simulink model "tensegrity_Val_like_sim_one_stage_v02"  (R2022b)
settings: Solver=ode15s  StartTime=0.0  StopTime=10  MaxStep=0.001  RelTol=1e-3
InitFcn:
  | tensegrity_Val_like_v02;
values from neighbouring files (symbols this model uses):
  a = 0.015    [parameters.m]
  A1 = [0.3, 0.3, 0.2]    [parameters_test_model.m]    (also in tensegrity_Val_like.m = [(G1+G2+G3)/3])
  A2 = [(G4+G5+G6)/3]    [tensegrity_Val_like.m]
  A3 = [(G7+G8+G9)/3]    [tensegrity_Val_like.m]
  A4 = [(B1+B2+B3)/3]    [tensegrity_Val_like.m]
  b_all = 2*ones(6, 1)    [parameters_test_model.m]
  F1 = [pos1(1), pos1(2), pos1(3)]    [parameters.m]
  F2 = [pos1(1)+dist, pos1(2), pos1(3)]    [parameters.m]
  F3 = [pos1(1)+dist/2, pos1(2)+dist, pos1(3)]    [parameters.m]
  F4 = [pos2(1), pos2(2), pos2(3)]    [parameters.m]
  F5 = [pos2(1)+dist, pos2(2), pos2(3)]    [parameters.m]
  F6 = [pos2(1)+dist/2, pos2(2)+dist, pos2(3)]    [parameters.m]
  F7 = [pos3(1), pos3(2), pos3(3)]    [parameters.m]
  F8 = [pos3(1)+dist, pos3(2), pos3(3)]    [parameters.m]
  F9 = [pos3(1)+dist/2, pos3(2)+dist, pos3(3)]    [parameters.m]
  k_all = 1e3*ones(6, 1)    [parameters_test_model.m]
  l = [0.08 0.08 0.08 0.15]'    [parameters.m]
  l0_all = [l01, l02, l03, l04, l05, l06]'    [parameters_test_model.m]
  lf = 0.05*ones(9, 1)    [parameters.m]
  predpeti = 0.95    [parameters_test_model.m]
undefined symbols (not defined in the file or in its folder): X, Y, Z
libraries: sm_lib x76, nesl_utility x73
(part 3 of 4)

== system tensegrity_Val_like_sim_one_stage_v02/internal cable force_19/cable force ==
  i : Inport
  Gain : Gain  Gain=predpeti
  PS-Simulink Converter1 : nesl_utility/PS-Simulink Converter  PhysicalDomain=network_engine_domain  SubClassName=ps_output  LeftPortType=input  RightPortType=output  PseudoPeriodic=off  Frequencies=[]  VectorFormat=1-D array  Unit=inherit  AffineConversion=off
  PS-Simulink Converter2 : nesl_utility/PS-Simulink Converter  PhysicalDomain=network_engine_domain  SubClassName=ps_output  LeftPortType=input  RightPortType=output  PseudoPeriodic=off  Frequencies=[]  VectorFormat=1-D array  Unit=inherit  AffineConversion=off
  Transform Sensor : sm_lib/Frames and Transforms/Transform Sensor  MeasurementFrame=World  SenseAngle=off  SenseAxis=off  SenseQ=off  SenseR=off  SenseRotationSequence=off  RotationSequence=XYX  SenseOmegaX=off  SenseOmegaY=off  SenseOmegaZ=off  SenseQDot=off  SenseRDot=off  SenseAlphaX=off  SenseAlphaY=off  SenseAlphaZ=off  SenseQDDot=off  SenseRDDot=off  SenseX=off  SenseY=off  SenseZ=off  SenseRad=off  SenseAzim=off  SenseDist=on  SenseInc=off  SenseXDot=off  SenseYDot=off  SenseZDot=off  SenseRadDot=off  SenseAzimDot=off  SenseDistDot=on  SenseIncDot=off  SenseXDDot=off  SenseYDDot=off  SenseZDDot=off  SenseRadDDot=off  SenseAzimDDot=off  SenseDistDDot=off  SenseIncDDot=off
  cable force computation : MATLAB Function  TreatAsAtomicUnit=on
  parameter selection : Subsystem
  TO : PMIOPort  Side=Right
  FROM : PMIOPort  Port=2  Side=Right
  Fc : Outport
  wires:
  Gain/1 -> cable force computation/3(l0)
  cable force computation/1(Fc) -> Fc/1
  parameter selection/2(b) -> cable force computation/2(b)
  parameter selection/3(l0) -> Gain/1
  parameter selection/1(k) -> cable force computation/1(k)
  PS-Simulink Converter1/1 -> cable force computation/4(l)
  PS-Simulink Converter2/1 -> cable force computation/5(v)
  i/1 -> parameter selection/1(i)
  connections:
  Transform Sensor/RConn3 -- PS-Simulink Converter2/LConn1
  Transform Sensor/RConn2 -- PS-Simulink Converter1/LConn1
  Transform Sensor/RConn1 -- TO/RConn1
  Transform Sensor/LConn1 -- FROM/RConn1

== system tensegrity_Val_like_sim_one_stage_v02/internal cable force_2/cable force ==
  i : Inport
  Gain : Gain  Gain=predpeti
  PS-Simulink Converter1 : nesl_utility/PS-Simulink Converter  PhysicalDomain=network_engine_domain  SubClassName=ps_output  LeftPortType=input  RightPortType=output  PseudoPeriodic=off  Frequencies=[]  VectorFormat=1-D array  Unit=inherit  AffineConversion=off
  PS-Simulink Converter2 : nesl_utility/PS-Simulink Converter  PhysicalDomain=network_engine_domain  SubClassName=ps_output  LeftPortType=input  RightPortType=output  PseudoPeriodic=off  Frequencies=[]  VectorFormat=1-D array  Unit=inherit  AffineConversion=off
  Transform Sensor : sm_lib/Frames and Transforms/Transform Sensor  MeasurementFrame=World  SenseAngle=off  SenseAxis=off  SenseQ=off  SenseR=off  SenseRotationSequence=off  RotationSequence=XYX  SenseOmegaX=off  SenseOmegaY=off  SenseOmegaZ=off  SenseQDot=off  SenseRDot=off  SenseAlphaX=off  SenseAlphaY=off  SenseAlphaZ=off  SenseQDDot=off  SenseRDDot=off  SenseX=off  SenseY=off  SenseZ=off  SenseRad=off  SenseAzim=off  SenseDist=on  SenseInc=off  SenseXDot=off  SenseYDot=off  SenseZDot=off  SenseRadDot=off  SenseAzimDot=off  SenseDistDot=on  SenseIncDot=off  SenseXDDot=off  SenseYDDot=off  SenseZDDot=off  SenseRadDDot=off  SenseAzimDDot=off  SenseDistDDot=off  SenseIncDDot=off
  cable force computation : MATLAB Function  TreatAsAtomicUnit=on
  parameter selection : Subsystem
  TO : PMIOPort  Side=Right
  FROM : PMIOPort  Port=2  Side=Right
  Fc : Outport
  wires:
  i/1 -> parameter selection/1(i)
  PS-Simulink Converter2/1 -> cable force computation/5(v)
  PS-Simulink Converter1/1 -> cable force computation/4(l)
  parameter selection/1(k) -> cable force computation/1(k)
  parameter selection/3(l0) -> Gain/1
  parameter selection/2(b) -> cable force computation/2(b)
  cable force computation/1(Fc) -> Fc/1
  Gain/1 -> cable force computation/3(l0)
  connections:
  Transform Sensor/LConn1 -- FROM/RConn1
  Transform Sensor/RConn1 -- TO/RConn1
  Transform Sensor/RConn2 -- PS-Simulink Converter1/LConn1
  Transform Sensor/RConn3 -- PS-Simulink Converter2/LConn1

== system tensegrity_Val_like_sim_one_stage_v02/internal cable force_20/cable force ==
  i : Inport
  Gain : Gain  Gain=predpeti
  PS-Simulink Converter1 : nesl_utility/PS-Simulink Converter  PhysicalDomain=network_engine_domain  SubClassName=ps_output  LeftPortType=input  RightPortType=output  PseudoPeriodic=off  Frequencies=[]  VectorFormat=1-D array  Unit=inherit  AffineConversion=off
  PS-Simulink Converter2 : nesl_utility/PS-Simulink Converter  PhysicalDomain=network_engine_domain  SubClassName=ps_output  LeftPortType=input  RightPortType=output  PseudoPeriodic=off  Frequencies=[]  VectorFormat=1-D array  Unit=inherit  AffineConversion=off
  Transform Sensor : sm_lib/Frames and Transforms/Transform Sensor  MeasurementFrame=World  SenseAngle=off  SenseAxis=off  SenseQ=off  SenseR=off  SenseRotationSequence=off  RotationSequence=XYX  SenseOmegaX=off  SenseOmegaY=off  SenseOmegaZ=off  SenseQDot=off  SenseRDot=off  SenseAlphaX=off  SenseAlphaY=off  SenseAlphaZ=off  SenseQDDot=off  SenseRDDot=off  SenseX=off  SenseY=off  SenseZ=off  SenseRad=off  SenseAzim=off  SenseDist=on  SenseInc=off  SenseXDot=off  SenseYDot=off  SenseZDot=off  SenseRadDot=off  SenseAzimDot=off  SenseDistDot=on  SenseIncDot=off  SenseXDDot=off  SenseYDDot=off  SenseZDDot=off  SenseRadDDot=off  SenseAzimDDot=off  SenseDistDDot=off  SenseIncDDot=off
  cable force computation : MATLAB Function  TreatAsAtomicUnit=on
  parameter selection : Subsystem
  TO : PMIOPort  Side=Right
  FROM : PMIOPort  Port=2  Side=Right
  Fc : Outport
  wires:
  i/1 -> parameter selection/1(i)
  PS-Simulink Converter2/1 -> cable force computation/5(v)
  PS-Simulink Converter1/1 -> cable force computation/4(l)
  parameter selection/1(k) -> cable force computation/1(k)
  parameter selection/3(l0) -> Gain/1
  parameter selection/2(b) -> cable force computation/2(b)
  cable force computation/1(Fc) -> Fc/1
  Gain/1 -> cable force computation/3(l0)
  connections:
  Transform Sensor/LConn1 -- FROM/RConn1
  Transform Sensor/RConn1 -- TO/RConn1
  Transform Sensor/RConn2 -- PS-Simulink Converter1/LConn1
  Transform Sensor/RConn3 -- PS-Simulink Converter2/LConn1

== system tensegrity_Val_like_sim_one_stage_v02/internal cable force_21/cable force ==
  i : Inport
  Gain : Gain  Gain=predpeti
  PS-Simulink Converter1 : nesl_utility/PS-Simulink Converter  PhysicalDomain=network_engine_domain  SubClassName=ps_output  LeftPortType=input  RightPortType=output  PseudoPeriodic=off  Frequencies=[]  VectorFormat=1-D array  Unit=inherit  AffineConversion=off
  PS-Simulink Converter2 : nesl_utility/PS-Simulink Converter  PhysicalDomain=network_engine_domain  SubClassName=ps_output  LeftPortType=input  RightPortType=output  PseudoPeriodic=off  Frequencies=[]  VectorFormat=1-D array  Unit=inherit  AffineConversion=off
  Transform Sensor : sm_lib/Frames and Transforms/Transform Sensor  MeasurementFrame=World  SenseAngle=off  SenseAxis=off  SenseQ=off  SenseR=off  SenseRotationSequence=off  RotationSequence=XYX  SenseOmegaX=off  SenseOmegaY=off  SenseOmegaZ=off  SenseQDot=off  SenseRDot=off  SenseAlphaX=off  SenseAlphaY=off  SenseAlphaZ=off  SenseQDDot=off  SenseRDDot=off  SenseX=off  SenseY=off  SenseZ=off  SenseRad=off  SenseAzim=off  SenseDist=on  SenseInc=off  SenseXDot=off  SenseYDot=off  SenseZDot=off  SenseRadDot=off  SenseAzimDot=off  SenseDistDot=on  SenseIncDot=off  SenseXDDot=off  SenseYDDot=off  SenseZDDot=off  SenseRadDDot=off  SenseAzimDDot=off  SenseDistDDot=off  SenseIncDDot=off
  cable force computation : MATLAB Function  TreatAsAtomicUnit=on
  parameter selection : Subsystem
  TO : PMIOPort  Side=Right
  FROM : PMIOPort  Port=2  Side=Right
  Fc : Outport
  wires:
  Gain/1 -> cable force computation/3(l0)
  cable force computation/1(Fc) -> Fc/1
  parameter selection/2(b) -> cable force computation/2(b)
  parameter selection/3(l0) -> Gain/1
  parameter selection/1(k) -> cable force computation/1(k)
  PS-Simulink Converter1/1 -> cable force computation/4(l)
  PS-Simulink Converter2/1 -> cable force computation/5(v)
  i/1 -> parameter selection/1(i)
  connections:
  Transform Sensor/RConn3 -- PS-Simulink Converter2/LConn1
  Transform Sensor/RConn2 -- PS-Simulink Converter1/LConn1
  Transform Sensor/RConn1 -- TO/RConn1
  Transform Sensor/LConn1 -- FROM/RConn1

== system tensegrity_Val_like_sim_one_stage_v02/internal cable force_22/cable force ==
  i : Inport
  Gain : Gain  Gain=predpeti
  PS-Simulink Converter1 : nesl_utility/PS-Simulink Converter  PhysicalDomain=network_engine_domain  SubClassName=ps_output  LeftPortType=input  RightPortType=output  PseudoPeriodic=off  Frequencies=[]  VectorFormat=1-D array  Unit=inherit  AffineConversion=off
  PS-Simulink Converter2 : nesl_utility/PS-Simulink Converter  PhysicalDomain=network_engine_domain  SubClassName=ps_output  LeftPortType=input  RightPortType=output  PseudoPeriodic=off  Frequencies=[]  VectorFormat=1-D array  Unit=inherit  AffineConversion=off
  Transform Sensor : sm_lib/Frames and Transforms/Transform Sensor  MeasurementFrame=World  SenseAngle=off  SenseAxis=off  SenseQ=off  SenseR=off  SenseRotationSequence=off  RotationSequence=XYX  SenseOmegaX=off  SenseOmegaY=off  SenseOmegaZ=off  SenseQDot=off  SenseRDot=off  SenseAlphaX=off  SenseAlphaY=off  SenseAlphaZ=off  SenseQDDot=off  SenseRDDot=off  SenseX=off  SenseY=off  SenseZ=off  SenseRad=off  SenseAzim=off  SenseDist=on  SenseInc=off  SenseXDot=off  SenseYDot=off  SenseZDot=off  SenseRadDot=off  SenseAzimDot=off  SenseDistDot=on  SenseIncDot=off  SenseXDDot=off  SenseYDDot=off  SenseZDDot=off  SenseRadDDot=off  SenseAzimDDot=off  SenseDistDDot=off  SenseIncDDot=off
  cable force computation : MATLAB Function  TreatAsAtomicUnit=on
  parameter selection : Subsystem
  TO : PMIOPort  Side=Right
  FROM : PMIOPort  Port=2  Side=Right
  Fc : Outport
  wires:
  Gain/1 -> cable force computation/3(l0)
  cable force computation/1(Fc) -> Fc/1
  parameter selection/2(b) -> cable force computation/2(b)
  parameter selection/3(l0) -> Gain/1
  parameter selection/1(k) -> cable force computation/1(k)
  PS-Simulink Converter1/1 -> cable force computation/4(l)
  PS-Simulink Converter2/1 -> cable force computation/5(v)
  i/1 -> parameter selection/1(i)
  connections:
  Transform Sensor/RConn3 -- PS-Simulink Converter2/LConn1
  Transform Sensor/RConn2 -- PS-Simulink Converter1/LConn1
  Transform Sensor/RConn1 -- TO/RConn1
  Transform Sensor/LConn1 -- FROM/RConn1

== system tensegrity_Val_like_sim_one_stage_v02/internal cable force_23/cable force ==
  i : Inport
  Gain : Gain  Gain=predpeti
  PS-Simulink Converter1 : nesl_utility/PS-Simulink Converter  PhysicalDomain=network_engine_domain  SubClassName=ps_output  LeftPortType=input  RightPortType=output  PseudoPeriodic=off  Frequencies=[]  VectorFormat=1-D array  Unit=inherit  AffineConversion=off
  PS-Simulink Converter2 : nesl_utility/PS-Simulink Converter  PhysicalDomain=network_engine_domain  SubClassName=ps_output  LeftPortType=input  RightPortType=output  PseudoPeriodic=off  Frequencies=[]  VectorFormat=1-D array  Unit=inherit  AffineConversion=off
  Transform Sensor : sm_lib/Frames and Transforms/Transform Sensor  MeasurementFrame=World  SenseAngle=off  SenseAxis=off  SenseQ=off  SenseR=off  SenseRotationSequence=off  RotationSequence=XYX  SenseOmegaX=off  SenseOmegaY=off  SenseOmegaZ=off  SenseQDot=off  SenseRDot=off  SenseAlphaX=off  SenseAlphaY=off  SenseAlphaZ=off  SenseQDDot=off  SenseRDDot=off  SenseX=off  SenseY=off  SenseZ=off  SenseRad=off  SenseAzim=off  SenseDist=on  SenseInc=off  SenseXDot=off  SenseYDot=off  SenseZDot=off  SenseRadDot=off  SenseAzimDot=off  SenseDistDot=on  SenseIncDot=off  SenseXDDot=off  SenseYDDot=off  SenseZDDot=off  SenseRadDDot=off  SenseAzimDDot=off  SenseDistDDot=off  SenseIncDDot=off
  cable force computation : MATLAB Function  TreatAsAtomicUnit=on
  parameter selection : Subsystem
  TO : PMIOPort  Side=Right
  FROM : PMIOPort  Port=2  Side=Right
  Fc : Outport
  wires:
  Gain/1 -> cable force computation/3(l0)
  cable force computation/1(Fc) -> Fc/1
  parameter selection/2(b) -> cable force computation/2(b)
  parameter selection/3(l0) -> Gain/1
  parameter selection/1(k) -> cable force computation/1(k)
  PS-Simulink Converter1/1 -> cable force computation/4(l)
  PS-Simulink Converter2/1 -> cable force computation/5(v)
  i/1 -> parameter selection/1(i)
  connections:
  Transform Sensor/RConn3 -- PS-Simulink Converter2/LConn1
  Transform Sensor/RConn2 -- PS-Simulink Converter1/LConn1
  Transform Sensor/RConn1 -- TO/RConn1
  Transform Sensor/LConn1 -- FROM/RConn1

== system tensegrity_Val_like_sim_one_stage_v02/internal cable force_3/cable force ==
  i : Inport
  Gain : Gain  Gain=predpeti
  PS-Simulink Converter1 : nesl_utility/PS-Simulink Converter  PhysicalDomain=network_engine_domain  SubClassName=ps_output  LeftPortType=input  RightPortType=output  PseudoPeriodic=off  Frequencies=[]  VectorFormat=1-D array  Unit=inherit  AffineConversion=off
  PS-Simulink Converter2 : nesl_utility/PS-Simulink Converter  PhysicalDomain=network_engine_domain  SubClassName=ps_output  LeftPortType=input  RightPortType=output  PseudoPeriodic=off  Frequencies=[]  VectorFormat=1-D array  Unit=inherit  AffineConversion=off
  Transform Sensor : sm_lib/Frames and Transforms/Transform Sensor  MeasurementFrame=World  SenseAngle=off  SenseAxis=off  SenseQ=off  SenseR=off  SenseRotationSequence=off  RotationSequence=XYX  SenseOmegaX=off  SenseOmegaY=off  SenseOmegaZ=off  SenseQDot=off  SenseRDot=off  SenseAlphaX=off  SenseAlphaY=off  SenseAlphaZ=off  SenseQDDot=off  SenseRDDot=off  SenseX=off  SenseY=off  SenseZ=off  SenseRad=off  SenseAzim=off  SenseDist=on  SenseInc=off  SenseXDot=off  SenseYDot=off  SenseZDot=off  SenseRadDot=off  SenseAzimDot=off  SenseDistDot=on  SenseIncDot=off  SenseXDDot=off  SenseYDDot=off  SenseZDDot=off  SenseRadDDot=off  SenseAzimDDot=off  SenseDistDDot=off  SenseIncDDot=off
  cable force computation : MATLAB Function  TreatAsAtomicUnit=on
  parameter selection : Subsystem
  TO : PMIOPort  Side=Right
  FROM : PMIOPort  Port=2  Side=Right
  Fc : Outport
  wires:
  Gain/1 -> cable force computation/3(l0)
  cable force computation/1(Fc) -> Fc/1
  parameter selection/2(b) -> cable force computation/2(b)
  parameter selection/3(l0) -> Gain/1
  parameter selection/1(k) -> cable force computation/1(k)
  PS-Simulink Converter1/1 -> cable force computation/4(l)
  PS-Simulink Converter2/1 -> cable force computation/5(v)
  i/1 -> parameter selection/1(i)
  connections:
  Transform Sensor/RConn3 -- PS-Simulink Converter2/LConn1
  Transform Sensor/RConn2 -- PS-Simulink Converter1/LConn1
  Transform Sensor/RConn1 -- TO/RConn1
  Transform Sensor/LConn1 -- FROM/RConn1

== system tensegrity_Val_like_sim_one_stage_v02/internal cable force_4/cable force ==
  i : Inport
  Gain : Gain  Gain=predpeti
  PS-Simulink Converter1 : nesl_utility/PS-Simulink Converter  PhysicalDomain=network_engine_domain  SubClassName=ps_output  LeftPortType=input  RightPortType=output  PseudoPeriodic=off  Frequencies=[]  VectorFormat=1-D array  Unit=inherit  AffineConversion=off
  PS-Simulink Converter2 : nesl_utility/PS-Simulink Converter  PhysicalDomain=network_engine_domain  SubClassName=ps_output  LeftPortType=input  RightPortType=output  PseudoPeriodic=off  Frequencies=[]  VectorFormat=1-D array  Unit=inherit  AffineConversion=off
  Transform Sensor : sm_lib/Frames and Transforms/Transform Sensor  MeasurementFrame=World  SenseAngle=off  SenseAxis=off  SenseQ=off  SenseR=off  SenseRotationSequence=off  RotationSequence=XYX  SenseOmegaX=off  SenseOmegaY=off  SenseOmegaZ=off  SenseQDot=off  SenseRDot=off  SenseAlphaX=off  SenseAlphaY=off  SenseAlphaZ=off  SenseQDDot=off  SenseRDDot=off  SenseX=off  SenseY=off  SenseZ=off  SenseRad=off  SenseAzim=off  SenseDist=on  SenseInc=off  SenseXDot=off  SenseYDot=off  SenseZDot=off  SenseRadDot=off  SenseAzimDot=off  SenseDistDot=on  SenseIncDot=off  SenseXDDot=off  SenseYDDot=off  SenseZDDot=off  SenseRadDDot=off  SenseAzimDDot=off  SenseDistDDot=off  SenseIncDDot=off
  cable force computation : MATLAB Function  TreatAsAtomicUnit=on
  parameter selection : Subsystem
  TO : PMIOPort  Side=Right
  FROM : PMIOPort  Port=2  Side=Right
  Fc : Outport
  wires:
  Gain/1 -> cable force computation/3(l0)
  cable force computation/1(Fc) -> Fc/1
  parameter selection/2(b) -> cable force computation/2(b)
  parameter selection/3(l0) -> Gain/1
  parameter selection/1(k) -> cable force computation/1(k)
  PS-Simulink Converter1/1 -> cable force computation/4(l)
  PS-Simulink Converter2/1 -> cable force computation/5(v)
  i/1 -> parameter selection/1(i)
  connections:
  Transform Sensor/RConn3 -- PS-Simulink Converter2/LConn1
  Transform Sensor/RConn2 -- PS-Simulink Converter1/LConn1
  Transform Sensor/RConn1 -- TO/RConn1
  Transform Sensor/LConn1 -- FROM/RConn1

== system tensegrity_Val_like_sim_one_stage_v02/internal cable force_5/cable force ==
  i : Inport
  Gain : Gain  Gain=predpeti
  PS-Simulink Converter1 : nesl_utility/PS-Simulink Converter  PhysicalDomain=network_engine_domain  SubClassName=ps_output  LeftPortType=input  RightPortType=output  PseudoPeriodic=off  Frequencies=[]  VectorFormat=1-D array  Unit=inherit  AffineConversion=off
  PS-Simulink Converter2 : nesl_utility/PS-Simulink Converter  PhysicalDomain=network_engine_domain  SubClassName=ps_output  LeftPortType=input  RightPortType=output  PseudoPeriodic=off  Frequencies=[]  VectorFormat=1-D array  Unit=inherit  AffineConversion=off
  Transform Sensor : sm_lib/Frames and Transforms/Transform Sensor  MeasurementFrame=World  SenseAngle=off  SenseAxis=off  SenseQ=off  SenseR=off  SenseRotationSequence=off  RotationSequence=XYX  SenseOmegaX=off  SenseOmegaY=off  SenseOmegaZ=off  SenseQDot=off  SenseRDot=off  SenseAlphaX=off  SenseAlphaY=off  SenseAlphaZ=off  SenseQDDot=off  SenseRDDot=off  SenseX=off  SenseY=off  SenseZ=off  SenseRad=off  SenseAzim=off  SenseDist=on  SenseInc=off  SenseXDot=off  SenseYDot=off  SenseZDot=off  SenseRadDot=off  SenseAzimDot=off  SenseDistDot=on  SenseIncDot=off  SenseXDDot=off  SenseYDDot=off  SenseZDDot=off  SenseRadDDot=off  SenseAzimDDot=off  SenseDistDDot=off  SenseIncDDot=off
  cable force computation : MATLAB Function  TreatAsAtomicUnit=on
  parameter selection : Subsystem
  TO : PMIOPort  Side=Right
  FROM : PMIOPort  Port=2  Side=Right
  Fc : Outport
  wires:
  i/1 -> parameter selection/1(i)
  PS-Simulink Converter2/1 -> cable force computation/5(v)
  PS-Simulink Converter1/1 -> cable force computation/4(l)
  parameter selection/1(k) -> cable force computation/1(k)
  parameter selection/3(l0) -> Gain/1
  parameter selection/2(b) -> cable force computation/2(b)
  cable force computation/1(Fc) -> Fc/1
  Gain/1 -> cable force computation/3(l0)
  connections:
  Transform Sensor/LConn1 -- FROM/RConn1
  Transform Sensor/RConn1 -- TO/RConn1
  Transform Sensor/RConn2 -- PS-Simulink Converter1/LConn1
  Transform Sensor/RConn3 -- PS-Simulink Converter2/LConn1

== system tensegrity_Val_like_sim_one_stage_v02/internal cable force_6/cable force ==
  i : Inport
  Gain : Gain  Gain=predpeti
  PS-Simulink Converter1 : nesl_utility/PS-Simulink Converter  PhysicalDomain=network_engine_domain  SubClassName=ps_output  LeftPortType=input  RightPortType=output  PseudoPeriodic=off  Frequencies=[]  VectorFormat=1-D array  Unit=inherit  AffineConversion=off
  PS-Simulink Converter2 : nesl_utility/PS-Simulink Converter  PhysicalDomain=network_engine_domain  SubClassName=ps_output  LeftPortType=input  RightPortType=output  PseudoPeriodic=off  Frequencies=[]  VectorFormat=1-D array  Unit=inherit  AffineConversion=off
  Transform Sensor : sm_lib/Frames and Transforms/Transform Sensor  MeasurementFrame=World  SenseAngle=off  SenseAxis=off  SenseQ=off  SenseR=off  SenseRotationSequence=off  RotationSequence=XYX  SenseOmegaX=off  SenseOmegaY=off  SenseOmegaZ=off  SenseQDot=off  SenseRDot=off  SenseAlphaX=off  SenseAlphaY=off  SenseAlphaZ=off  SenseQDDot=off  SenseRDDot=off  SenseX=off  SenseY=off  SenseZ=off  SenseRad=off  SenseAzim=off  SenseDist=on  SenseInc=off  SenseXDot=off  SenseYDot=off  SenseZDot=off  SenseRadDot=off  SenseAzimDot=off  SenseDistDot=on  SenseIncDot=off  SenseXDDot=off  SenseYDDot=off  SenseZDDot=off  SenseRadDDot=off  SenseAzimDDot=off  SenseDistDDot=off  SenseIncDDot=off
  cable force computation : MATLAB Function  TreatAsAtomicUnit=on
  parameter selection : Subsystem
  TO : PMIOPort  Side=Right
  FROM : PMIOPort  Port=2  Side=Right
  Fc : Outport
  wires:
  Gain/1 -> cable force computation/3(l0)
  cable force computation/1(Fc) -> Fc/1
  parameter selection/2(b) -> cable force computation/2(b)
  parameter selection/3(l0) -> Gain/1
  parameter selection/1(k) -> cable force computation/1(k)
  PS-Simulink Converter1/1 -> cable force computation/4(l)
  PS-Simulink Converter2/1 -> cable force computation/5(v)
  i/1 -> parameter selection/1(i)
  connections:
  Transform Sensor/RConn3 -- PS-Simulink Converter2/LConn1
  Transform Sensor/RConn2 -- PS-Simulink Converter1/LConn1
  Transform Sensor/RConn1 -- TO/RConn1
  Transform Sensor/LConn1 -- FROM/RConn1

== system tensegrity_Val_like_sim_one_stage_v02/internal cable force_7/cable force ==
  i : Inport
  Gain : Gain  Gain=predpeti
  PS-Simulink Converter1 : nesl_utility/PS-Simulink Converter  PhysicalDomain=network_engine_domain  SubClassName=ps_output  LeftPortType=input  RightPortType=output  PseudoPeriodic=off  Frequencies=[]  VectorFormat=1-D array  Unit=inherit  AffineConversion=off
  PS-Simulink Converter2 : nesl_utility/PS-Simulink Converter  PhysicalDomain=network_engine_domain  SubClassName=ps_output  LeftPortType=input  RightPortType=output  PseudoPeriodic=off  Frequencies=[]  VectorFormat=1-D array  Unit=inherit  AffineConversion=off
  Transform Sensor : sm_lib/Frames and Transforms/Transform Sensor  MeasurementFrame=World  SenseAngle=off  SenseAxis=off  SenseQ=off  SenseR=off  SenseRotationSequence=off  RotationSequence=XYX  SenseOmegaX=off  SenseOmegaY=off  SenseOmegaZ=off  SenseQDot=off  SenseRDot=off  SenseAlphaX=off  SenseAlphaY=off  SenseAlphaZ=off  SenseQDDot=off  SenseRDDot=off  SenseX=off  SenseY=off  SenseZ=off  SenseRad=off  SenseAzim=off  SenseDist=on  SenseInc=off  SenseXDot=off  SenseYDot=off  SenseZDot=off  SenseRadDot=off  SenseAzimDot=off  SenseDistDot=on  SenseIncDot=off  SenseXDDot=off  SenseYDDot=off  SenseZDDot=off  SenseRadDDot=off  SenseAzimDDot=off  SenseDistDDot=off  SenseIncDDot=off
  cable force computation : MATLAB Function  TreatAsAtomicUnit=on
  parameter selection : Subsystem
  TO : PMIOPort  Side=Right
  FROM : PMIOPort  Port=2  Side=Right
  Fc : Outport
  wires:
  Gain/1 -> cable force computation/3(l0)
  cable force computation/1(Fc) -> Fc/1
  parameter selection/2(b) -> cable force computation/2(b)
  parameter selection/3(l0) -> Gain/1
  parameter selection/1(k) -> cable force computation/1(k)
  PS-Simulink Converter1/1 -> cable force computation/4(l)
  PS-Simulink Converter2/1 -> cable force computation/5(v)
  i/1 -> parameter selection/1(i)
  connections:
  Transform Sensor/RConn3 -- PS-Simulink Converter2/LConn1
  Transform Sensor/RConn2 -- PS-Simulink Converter1/LConn1
  Transform Sensor/RConn1 -- TO/RConn1
  Transform Sensor/LConn1 -- FROM/RConn1

== system tensegrity_Val_like_sim_one_stage_v02/internal cable force_8/cable force ==
  i : Inport
  Gain : Gain  Gain=predpeti
  PS-Simulink Converter1 : nesl_utility/PS-Simulink Converter  PhysicalDomain=network_engine_domain  SubClassName=ps_output  LeftPortType=input  RightPortType=output  PseudoPeriodic=off  Frequencies=[]  VectorFormat=1-D array  Unit=inherit  AffineConversion=off
  PS-Simulink Converter2 : nesl_utility/PS-Simulink Converter  PhysicalDomain=network_engine_domain  SubClassName=ps_output  LeftPortType=input  RightPortType=output  PseudoPeriodic=off  Frequencies=[]  VectorFormat=1-D array  Unit=inherit  AffineConversion=off
  Transform Sensor : sm_lib/Frames and Transforms/Transform Sensor  MeasurementFrame=World  SenseAngle=off  SenseAxis=off  SenseQ=off  SenseR=off  SenseRotationSequence=off  RotationSequence=XYX  SenseOmegaX=off  SenseOmegaY=off  SenseOmegaZ=off  SenseQDot=off  SenseRDot=off  SenseAlphaX=off  SenseAlphaY=off  SenseAlphaZ=off  SenseQDDot=off  SenseRDDot=off  SenseX=off  SenseY=off  SenseZ=off  SenseRad=off  SenseAzim=off  SenseDist=on  SenseInc=off  SenseXDot=off  SenseYDot=off  SenseZDot=off  SenseRadDot=off  SenseAzimDot=off  SenseDistDot=on  SenseIncDot=off  SenseXDDot=off  SenseYDDot=off  SenseZDDot=off  SenseRadDDot=off  SenseAzimDDot=off  SenseDistDDot=off  SenseIncDDot=off
  cable force computation : MATLAB Function  TreatAsAtomicUnit=on
  parameter selection : Subsystem
  TO : PMIOPort  Side=Right
  FROM : PMIOPort  Port=2  Side=Right
  Fc : Outport
  wires:
  i/1 -> parameter selection/1(i)
  PS-Simulink Converter2/1 -> cable force computation/5(v)
  PS-Simulink Converter1/1 -> cable force computation/4(l)
  parameter selection/1(k) -> cable force computation/1(k)
  parameter selection/3(l0) -> Gain/1
  parameter selection/2(b) -> cable force computation/2(b)
  cable force computation/1(Fc) -> Fc/1
  Gain/1 -> cable force computation/3(l0)
  connections:
  Transform Sensor/LConn1 -- FROM/RConn1
  Transform Sensor/RConn1 -- TO/RConn1
  Transform Sensor/RConn2 -- PS-Simulink Converter1/LConn1
  Transform Sensor/RConn3 -- PS-Simulink Converter2/LConn1

== system tensegrity_Val_like_sim_one_stage_v02/internal cable force_9/cable force ==
  i : Inport
  Gain : Gain  Gain=predpeti
  PS-Simulink Converter1 : nesl_utility/PS-Simulink Converter  PhysicalDomain=network_engine_domain  SubClassName=ps_output  LeftPortType=input  RightPortType=output  PseudoPeriodic=off  Frequencies=[]  VectorFormat=1-D array  Unit=inherit  AffineConversion=off
  PS-Simulink Converter2 : nesl_utility/PS-Simulink Converter  PhysicalDomain=network_engine_domain  SubClassName=ps_output  LeftPortType=input  RightPortType=output  PseudoPeriodic=off  Frequencies=[]  VectorFormat=1-D array  Unit=inherit  AffineConversion=off
  Transform Sensor : sm_lib/Frames and Transforms/Transform Sensor  MeasurementFrame=World  SenseAngle=off  SenseAxis=off  SenseQ=off  SenseR=off  SenseRotationSequence=off  RotationSequence=XYX  SenseOmegaX=off  SenseOmegaY=off  SenseOmegaZ=off  SenseQDot=off  SenseRDot=off  SenseAlphaX=off  SenseAlphaY=off  SenseAlphaZ=off  SenseQDDot=off  SenseRDDot=off  SenseX=off  SenseY=off  SenseZ=off  SenseRad=off  SenseAzim=off  SenseDist=on  SenseInc=off  SenseXDot=off  SenseYDot=off  SenseZDot=off  SenseRadDot=off  SenseAzimDot=off  SenseDistDot=on  SenseIncDot=off  SenseXDDot=off  SenseYDDot=off  SenseZDDot=off  SenseRadDDot=off  SenseAzimDDot=off  SenseDistDDot=off  SenseIncDDot=off
  cable force computation : MATLAB Function  TreatAsAtomicUnit=on
  parameter selection : Subsystem
  TO : PMIOPort  Side=Right
  FROM : PMIOPort  Port=2  Side=Right
  Fc : Outport
  wires:
  Gain/1 -> cable force computation/3(l0)
  cable force computation/1(Fc) -> Fc/1
  parameter selection/2(b) -> cable force computation/2(b)
  parameter selection/3(l0) -> Gain/1
  parameter selection/1(k) -> cable force computation/1(k)
  PS-Simulink Converter1/1 -> cable force computation/4(l)
  PS-Simulink Converter2/1 -> cable force computation/5(v)
  i/1 -> parameter selection/1(i)
  connections:
  Transform Sensor/RConn3 -- PS-Simulink Converter2/LConn1
  Transform Sensor/RConn2 -- PS-Simulink Converter1/LConn1
  Transform Sensor/RConn1 -- TO/RConn1
  Transform Sensor/LConn1 -- FROM/RConn1

== system tensegrity_Val_like_sim_one_stage_v02/internal cable force_1/cable force/parameter selection ==
  i : Inport
  damping : Constant  Value=b_all
  free length : Constant  Value=l0_all
  parameter selection : MATLAB Function  TreatAsAtomicUnit=on
  stiffness : Constant  Value=k_all
  k : Outport
  b : Outport  Port=2
  l0 : Outport  Port=3
  wires:
  damping/1 -> parameter selection/3(b_all)
  stiffness/1 -> parameter selection/2(k_all)
  free length/1 -> parameter selection/4(l0_all)
  parameter selection/2(b) -> b/1
  i/1 -> parameter selection/1(i)
  parameter selection/3(l0) -> l0/1
  parameter selection/1(k) -> k/1

== system tensegrity_Val_like_sim_one_stage_v02/internal cable force_10/cable force/parameter selection ==
  i : Inport
  damping : Constant  Value=b_all
  free length : Constant  Value=l0_all
  parameter selection : MATLAB Function  TreatAsAtomicUnit=on
  stiffness : Constant  Value=k_all
  k : Outport
  b : Outport  Port=2
  l0 : Outport  Port=3
  wires:
  damping/1 -> parameter selection/3(b_all)
  stiffness/1 -> parameter selection/2(k_all)
  free length/1 -> parameter selection/4(l0_all)
  parameter selection/2(b) -> b/1
  i/1 -> parameter selection/1(i)
  parameter selection/3(l0) -> l0/1
  parameter selection/1(k) -> k/1

== system tensegrity_Val_like_sim_one_stage_v02/internal cable force_11/cable force/parameter selection ==
  i : Inport
  damping : Constant  Value=b_all
  free length : Constant  Value=l0_all
  parameter selection : MATLAB Function  TreatAsAtomicUnit=on
  stiffness : Constant  Value=k_all
  k : Outport
  b : Outport  Port=2
  l0 : Outport  Port=3
  wires:
  parameter selection/1(k) -> k/1
  parameter selection/3(l0) -> l0/1
  i/1 -> parameter selection/1(i)
  parameter selection/2(b) -> b/1
  free length/1 -> parameter selection/4(l0_all)
  stiffness/1 -> parameter selection/2(k_all)
  damping/1 -> parameter selection/3(b_all)

== system tensegrity_Val_like_sim_one_stage_v02/internal cable force_12/cable force/parameter selection ==
  i : Inport
  damping : Constant  Value=b_all
  free length : Constant  Value=l0_all
  parameter selection : MATLAB Function  TreatAsAtomicUnit=on
  stiffness : Constant  Value=k_all
  k : Outport
  b : Outport  Port=2
  l0 : Outport  Port=3
  wires:
  damping/1 -> parameter selection/3(b_all)
  stiffness/1 -> parameter selection/2(k_all)
  free length/1 -> parameter selection/4(l0_all)
  parameter selection/2(b) -> b/1
  i/1 -> parameter selection/1(i)
  parameter selection/3(l0) -> l0/1
  parameter selection/1(k) -> k/1

== system tensegrity_Val_like_sim_one_stage_v02/internal cable force_120/cable force/parameter selection ==
  i : Inport
  damping : Constant  Value=b_all
  free length : Constant  Value=l0_all
  parameter selection : MATLAB Function  TreatAsAtomicUnit=on
  stiffness : Constant  Value=k_all
  k : Outport
  b : Outport  Port=2
  l0 : Outport  Port=3
  wires:
  parameter selection/1(k) -> k/1
  parameter selection/3(l0) -> l0/1
  i/1 -> parameter selection/1(i)
  parameter selection/2(b) -> b/1
  free length/1 -> parameter selection/4(l0_all)
  stiffness/1 -> parameter selection/2(k_all)
  damping/1 -> parameter selection/3(b_all)

== system tensegrity_Val_like_sim_one_stage_v02/internal cable force_13/cable force/parameter selection ==
  i : Inport
  damping : Constant  Value=b_all
  free length : Constant  Value=l0_all
  parameter selection : MATLAB Function  TreatAsAtomicUnit=on
  stiffness : Constant  Value=k_all
  k : Outport
  b : Outport  Port=2
  l0 : Outport  Port=3
  wires:
  damping/1 -> parameter selection/3(b_all)
  stiffness/1 -> parameter selection/2(k_all)
  free length/1 -> parameter selection/4(l0_all)
  parameter selection/2(b) -> b/1
  i/1 -> parameter selection/1(i)
  parameter selection/3(l0) -> l0/1
  parameter selection/1(k) -> k/1

== system tensegrity_Val_like_sim_one_stage_v02/internal cable force_14/cable force/parameter selection ==
  i : Inport
  damping : Constant  Value=b_all
  free length : Constant  Value=l0_all
  parameter selection : MATLAB Function  TreatAsAtomicUnit=on
  stiffness : Constant  Value=k_all
  k : Outport
  b : Outport  Port=2
  l0 : Outport  Port=3
  wires:
  parameter selection/1(k) -> k/1
  parameter selection/3(l0) -> l0/1
  i/1 -> parameter selection/1(i)
  parameter selection/2(b) -> b/1
  free length/1 -> parameter selection/4(l0_all)
  stiffness/1 -> parameter selection/2(k_all)
  damping/1 -> parameter selection/3(b_all)

== system tensegrity_Val_like_sim_one_stage_v02/internal cable force_15/cable force/parameter selection ==
  i : Inport
  damping : Constant  Value=b_all
  free length : Constant  Value=l0_all
  parameter selection : MATLAB Function  TreatAsAtomicUnit=on
  stiffness : Constant  Value=k_all
  k : Outport
  b : Outport  Port=2
  l0 : Outport  Port=3
  wires:
  damping/1 -> parameter selection/3(b_all)
  stiffness/1 -> parameter selection/2(k_all)
  free length/1 -> parameter selection/4(l0_all)
  parameter selection/2(b) -> b/1
  i/1 -> parameter selection/1(i)
  parameter selection/3(l0) -> l0/1
  parameter selection/1(k) -> k/1

== system tensegrity_Val_like_sim_one_stage_v02/internal cable force_16/cable force/parameter selection ==
  i : Inport
  damping : Constant  Value=b_all
  free length : Constant  Value=l0_all
  parameter selection : MATLAB Function  TreatAsAtomicUnit=on
  stiffness : Constant  Value=k_all
  k : Outport
  b : Outport  Port=2
  l0 : Outport  Port=3
  wires:
  damping/1 -> parameter selection/3(b_all)
  stiffness/1 -> parameter selection/2(k_all)
  free length/1 -> parameter selection/4(l0_all)
  parameter selection/2(b) -> b/1
  i/1 -> parameter selection/1(i)
  parameter selection/3(l0) -> l0/1
  parameter selection/1(k) -> k/1

== system tensegrity_Val_like_sim_one_stage_v02/internal cable force_17/cable force/parameter selection ==
  i : Inport
  damping : Constant  Value=b_all
  free length : Constant  Value=l0_all
  parameter selection : MATLAB Function  TreatAsAtomicUnit=on
  stiffness : Constant  Value=k_all
  k : Outport
  b : Outport  Port=2
  l0 : Outport  Port=3
  wires:
  parameter selection/1(k) -> k/1
  parameter selection/3(l0) -> l0/1
  i/1 -> parameter selection/1(i)
  parameter selection/2(b) -> b/1
  free length/1 -> parameter selection/4(l0_all)
  stiffness/1 -> parameter selection/2(k_all)
  damping/1 -> parameter selection/3(b_all)

== system tensegrity_Val_like_sim_one_stage_v02/internal cable force_18/cable force/parameter selection ==
  i : Inport
  damping : Constant  Value=b_all
  free length : Constant  Value=l0_all
  parameter selection : MATLAB Function  TreatAsAtomicUnit=on
  stiffness : Constant  Value=k_all
  k : Outport
  b : Outport  Port=2
  l0 : Outport  Port=3
  wires:
  damping/1 -> parameter selection/3(b_all)
  stiffness/1 -> parameter selection/2(k_all)
  free length/1 -> parameter selection/4(l0_all)
  parameter selection/2(b) -> b/1
  i/1 -> parameter selection/1(i)
  parameter selection/3(l0) -> l0/1
  parameter selection/1(k) -> k/1

== system tensegrity_Val_like_sim_one_stage_v02/internal cable force_19/cable force/parameter selection ==
  i : Inport
  damping : Constant  Value=b_all
  free length : Constant  Value=l0_all
  parameter selection : MATLAB Function  TreatAsAtomicUnit=on
  stiffness : Constant  Value=k_all
  k : Outport
  b : Outport  Port=2
  l0 : Outport  Port=3
  wires:
  damping/1 -> parameter selection/3(b_all)
  stiffness/1 -> parameter selection/2(k_all)
  free length/1 -> parameter selection/4(l0_all)
  parameter selection/2(b) -> b/1
  i/1 -> parameter selection/1(i)
  parameter selection/3(l0) -> l0/1
  parameter selection/1(k) -> k/1

== system tensegrity_Val_like_sim_one_stage_v02/internal cable force_2/cable force/parameter selection ==
  i : Inport
  damping : Constant  Value=b_all
  free length : Constant  Value=l0_all
  parameter selection : MATLAB Function  TreatAsAtomicUnit=on
  stiffness : Constant  Value=k_all
  k : Outport
  b : Outport  Port=2
  l0 : Outport  Port=3
  wires:
  parameter selection/1(k) -> k/1
  parameter selection/3(l0) -> l0/1
  i/1 -> parameter selection/1(i)
  parameter selection/2(b) -> b/1
  free length/1 -> parameter selection/4(l0_all)
  stiffness/1 -> parameter selection/2(k_all)
  damping/1 -> parameter selection/3(b_all)

== system tensegrity_Val_like_sim_one_stage_v02/internal cable force_20/cable force/parameter selection ==
  i : Inport
  damping : Constant  Value=b_all
  free length : Constant  Value=l0_all
  parameter selection : MATLAB Function  TreatAsAtomicUnit=on
  stiffness : Constant  Value=k_all
  k : Outport
  b : Outport  Port=2
  l0 : Outport  Port=3
  wires:
  parameter selection/1(k) -> k/1
  parameter selection/3(l0) -> l0/1
  i/1 -> parameter selection/1(i)
  parameter selection/2(b) -> b/1
  free length/1 -> parameter selection/4(l0_all)
  stiffness/1 -> parameter selection/2(k_all)
  damping/1 -> parameter selection/3(b_all)

== system tensegrity_Val_like_sim_one_stage_v02/internal cable force_21/cable force/parameter selection ==
  i : Inport
  damping : Constant  Value=b_all
  free length : Constant  Value=l0_all
  parameter selection : MATLAB Function  TreatAsAtomicUnit=on
  stiffness : Constant  Value=k_all
  k : Outport
  b : Outport  Port=2
  l0 : Outport  Port=3
  wires:
  damping/1 -> parameter selection/3(b_all)
  stiffness/1 -> parameter selection/2(k_all)
  free length/1 -> parameter selection/4(l0_all)
  parameter selection/2(b) -> b/1
  i/1 -> parameter selection/1(i)
  parameter selection/3(l0) -> l0/1
  parameter selection/1(k) -> k/1

== system tensegrity_Val_like_sim_one_stage_v02/internal cable force_22/cable force/parameter selection ==
  i : Inport
  damping : Constant  Value=b_all
  free length : Constant  Value=l0_all
  parameter selection : MATLAB Function  TreatAsAtomicUnit=on
  stiffness : Constant  Value=k_all
  k : Outport
  b : Outport  Port=2
  l0 : Outport  Port=3
  wires:
  damping/1 -> parameter selection/3(b_all)
  stiffness/1 -> parameter selection/2(k_all)
  free length/1 -> parameter selection/4(l0_all)
  parameter selection/2(b) -> b/1
  i/1 -> parameter selection/1(i)
  parameter selection/3(l0) -> l0/1
  parameter selection/1(k) -> k/1

== system tensegrity_Val_like_sim_one_stage_v02/internal cable force_23/cable force/parameter selection ==
  i : Inport
  damping : Constant  Value=b_all
  free length : Constant  Value=l0_all
  parameter selection : MATLAB Function  TreatAsAtomicUnit=on
  stiffness : Constant  Value=k_all
  k : Outport
  b : Outport  Port=2
  l0 : Outport  Port=3
  wires:
  damping/1 -> parameter selection/3(b_all)
  stiffness/1 -> parameter selection/2(k_all)
  free length/1 -> parameter selection/4(l0_all)
  parameter selection/2(b) -> b/1
  i/1 -> parameter selection/1(i)
  parameter selection/3(l0) -> l0/1
  parameter selection/1(k) -> k/1

== system tensegrity_Val_like_sim_one_stage_v02/internal cable force_3/cable force/parameter selection ==
  i : Inport
  damping : Constant  Value=b_all
  free length : Constant  Value=l0_all
  parameter selection : MATLAB Function  TreatAsAtomicUnit=on
  stiffness : Constant  Value=k_all
  k : Outport
  b : Outport  Port=2
  l0 : Outport  Port=3
  wires:
  damping/1 -> parameter selection/3(b_all)
  stiffness/1 -> parameter selection/2(k_all)
  free length/1 -> parameter selection/4(l0_all)
  parameter selection/2(b) -> b/1
  i/1 -> parameter selection/1(i)
  parameter selection/3(l0) -> l0/1
  parameter selection/1(k) -> k/1

== system tensegrity_Val_like_sim_one_stage_v02/internal cable force_4/cable force/parameter selection ==
  i : Inport
  damping : Constant  Value=b_all
  free length : Constant  Value=l0_all
  parameter selection : MATLAB Function  TreatAsAtomicUnit=on
  stiffness : Constant  Value=k_all
  k : Outport
  b : Outport  Port=2
  l0 : Outport  Port=3
  wires:
  damping/1 -> parameter selection/3(b_all)
  stiffness/1 -> parameter selection/2(k_all)
  free length/1 -> parameter selection/4(l0_all)
  parameter selection/2(b) -> b/1
  i/1 -> parameter selection/1(i)
  parameter selection/3(l0) -> l0/1
  parameter selection/1(k) -> k/1

== system tensegrity_Val_like_sim_one_stage_v02/internal cable force_5/cable force/parameter selection ==
  i : Inport
  damping : Constant  Value=b_all
  free length : Constant  Value=l0_all
  parameter selection : MATLAB Function  TreatAsAtomicUnit=on
  stiffness : Constant  Value=k_all
  k : Outport
  b : Outport  Port=2
  l0 : Outport  Port=3
  wires:
  parameter selection/1(k) -> k/1
  parameter selection/3(l0) -> l0/1
  i/1 -> parameter selection/1(i)
  parameter selection/2(b) -> b/1
  free length/1 -> parameter selection/4(l0_all)
  stiffness/1 -> parameter selection/2(k_all)
  damping/1 -> parameter selection/3(b_all)

== system tensegrity_Val_like_sim_one_stage_v02/internal cable force_6/cable force/parameter selection ==
  i : Inport
  damping : Constant  Value=b_all
  free length : Constant  Value=l0_all
  parameter selection : MATLAB Function  TreatAsAtomicUnit=on
  stiffness : Constant  Value=k_all
  k : Outport
  b : Outport  Port=2
  l0 : Outport  Port=3
  wires:
  damping/1 -> parameter selection/3(b_all)
  stiffness/1 -> parameter selection/2(k_all)
  free length/1 -> parameter selection/4(l0_all)
  parameter selection/2(b) -> b/1
  i/1 -> parameter selection/1(i)
  parameter selection/3(l0) -> l0/1
  parameter selection/1(k) -> k/1

== system tensegrity_Val_like_sim_one_stage_v02/internal cable force_7/cable force/parameter selection ==
  i : Inport
  damping : Constant  Value=b_all
  free length : Constant  Value=l0_all
  parameter selection : MATLAB Function  TreatAsAtomicUnit=on
  stiffness : Constant  Value=k_all
  k : Outport
  b : Outport  Port=2
  l0 : Outport  Port=3
  wires:
  damping/1 -> parameter selection/3(b_all)
  stiffness/1 -> parameter selection/2(k_all)
  free length/1 -> parameter selection/4(l0_all)
  parameter selection/2(b) -> b/1
  i/1 -> parameter selection/1(i)
  parameter selection/3(l0) -> l0/1
  parameter selection/1(k) -> k/1

== system tensegrity_Val_like_sim_one_stage_v02/internal cable force_8/cable force/parameter selection ==
  i : Inport
  damping : Constant  Value=b_all
  free length : Constant  Value=l0_all
  parameter selection : MATLAB Function  TreatAsAtomicUnit=on
  stiffness : Constant  Value=k_all
  k : Outport
  b : Outport  Port=2
  l0 : Outport  Port=3
  wires:
  parameter selection/1(k) -> k/1
  parameter selection/3(l0) -> l0/1
  i/1 -> parameter selection/1(i)
  parameter selection/2(b) -> b/1
  free length/1 -> parameter selection/4(l0_all)
  stiffness/1 -> parameter selection/2(k_all)
  damping/1 -> parameter selection/3(b_all)

== system tensegrity_Val_like_sim_one_stage_v02/internal cable force_9/cable force/parameter selection ==
  i : Inport
  damping : Constant  Value=b_all
  free length : Constant  Value=l0_all
  parameter selection : MATLAB Function  TreatAsAtomicUnit=on
  stiffness : Constant  Value=k_all
  k : Outport
  b : Outport  Port=2
  l0 : Outport  Port=3
  wires:
  damping/1 -> parameter selection/3(b_all)
  stiffness/1 -> parameter selection/2(k_all)
  free length/1 -> parameter selection/4(l0_all)
  parameter selection/2(b) -> b/1
  i/1 -> parameter selection/1(i)
  parameter selection/3(l0) -> l0/1
  parameter selection/1(k) -> k/1

== matlab function tensegrity_Val_like_sim_one_stage_v02/internal cable force_6/cable force/cable force computation ==
  data: k input; Fc output; b input; l0 input; l input; v input
function Fc = cable_force(k, b,l0, l, v)

Fc=k*(l-l0) + b*v;

== matlab function tensegrity_Val_like_sim_one_stage_v02/internal cable force_6/cable force/parameter selection/parameter selection ==
  data: i input; k output; k_all input; b_all input; l0_all input; b output; l0 output
function [k, b, l0] = parameter_selection(i, k_all, b_all, l0_all)

k=k_all(i);
b=b_all(i);
l0=l0_all(i);

== matlab function tensegrity_Val_like_sim_one_stage_v02/internal cable force_2/cable force/cable force computation ==
  data: k input; Fc output; b input; l0 input; l input; v input
function Fc = cable_force(k, b,l0, l, v)

Fc=k*(l-l0) + b*v;

== matlab function tensegrity_Val_like_sim_one_stage_v02/internal cable force_10/cable force/cable force computation ==
  data: k input; Fc output; b input; l0 input; l input; v input
function Fc = cable_force(k, b,l0, l, v)

Fc=k*(l-l0) + b*v;

== matlab function tensegrity_Val_like_sim_one_stage_v02/internal cable force_10/cable force/parameter selection/parameter selection ==
  data: i input; k output; k_all input; b_all input; l0_all input; b output; l0 output
function [k, b, l0] = parameter_selection(i, k_all, b_all, l0_all)

k=k_all(i);
b=b_all(i);
l0=l0_all(i);

== matlab function tensegrity_Val_like_sim_one_stage_v02/internal cable force_1/cable force/cable force computation ==
  data: k input; Fc output; b input; l0 input; l input; v input
function Fc = cable_force(k, b,l0, l, v)

Fc=k*(l-l0) + b*v;

== matlab function tensegrity_Val_like_sim_one_stage_v02/internal cable force_1/cable force/parameter selection/parameter selection ==
  data: i input; k output; k_all input; b_all input; l0_all input; b output; l0 output
function [k, b, l0] = parameter_selection(i, k_all, b_all, l0_all)

k=k_all(i);
b=b_all(i);
l0=l0_all(i);

== matlab function tensegrity_Val_like_sim_one_stage_v02/internal cable force_11/cable force/cable force computation ==
  data: k input; Fc output; b input; l0 input; l input; v input
function Fc = cable_force(k, b,l0, l, v)

Fc=k*(l-l0) + b*v;

== matlab function tensegrity_Val_like_sim_one_stage_v02/internal cable force_11/cable force/parameter selection/parameter selection ==
  data: i input; k output; k_all input; b_all input; l0_all input; b output; l0 output
function [k, b, l0] = parameter_selection(i, k_all, b_all, l0_all)

k=k_all(i);
b=b_all(i);
l0=l0_all(i);

== matlab function tensegrity_Val_like_sim_one_stage_v02/internal cable force_12/cable force/cable force computation ==
  data: k input; Fc output; b input; l0 input; l input; v input
function Fc = cable_force(k, b,l0, l, v)

Fc=k*(l-l0) + b*v;

== matlab function tensegrity_Val_like_sim_one_stage_v02/internal cable force_12/cable force/parameter selection/parameter selection ==
  data: i input; k output; k_all input; b_all input; l0_all input; b output; l0 output
function [k, b, l0] = parameter_selection(i, k_all, b_all, l0_all)

k=k_all(i);
b=b_all(i);
l0=l0_all(i);

== matlab function tensegrity_Val_like_sim_one_stage_v02/internal cable force_7/cable force/cable force computation ==
  data: k input; Fc output; b input; l0 input; l input; v input
function Fc = cable_force(k, b,l0, l, v)

Fc=k*(l-l0) + b*v;

== matlab function tensegrity_Val_like_sim_one_stage_v02/internal cable force_2/cable force/parameter selection/parameter selection ==
  data: i input; k output; k_all input; b_all input; l0_all input; b output; l0 output
function [k, b, l0] = parameter_selection(i, k_all, b_all, l0_all)

k=k_all(i);
b=b_all(i);
l0=l0_all(i);

== matlab function tensegrity_Val_like_sim_one_stage_v02/internal cable force_7/cable force/parameter selection/parameter selection ==
  data: i input; k output; k_all input; b_all input; l0_all input; b output; l0 output
function [k, b, l0] = parameter_selection(i, k_all, b_all, l0_all)

k=k_all(i);
b=b_all(i);
l0=l0_all(i);

== matlab function tensegrity_Val_like_sim_one_stage_v02/internal cable force_8/cable force/cable force computation ==
  data: k input; Fc output; b input; l0 input; l input; v input
function Fc = cable_force(k, b,l0, l, v)

Fc=k*(l-l0) + b*v;

== matlab function tensegrity_Val_like_sim_one_stage_v02/internal cable force_8/cable force/parameter selection/parameter selection ==
  data: i input; k output; k_all input; b_all input; l0_all input; b output; l0 output
function [k, b, l0] = parameter_selection(i, k_all, b_all, l0_all)

k=k_all(i);
b=b_all(i);
l0=l0_all(i);

== matlab function tensegrity_Val_like_sim_one_stage_v02/internal cable force_9/cable force/cable force computation ==
  data: k input; Fc output; b input; l0 input; l input; v input
function Fc = cable_force(k, b,l0, l, v)

Fc=k*(l-l0) + b*v;

== matlab function tensegrity_Val_like_sim_one_stage_v02/internal cable force_9/cable force/parameter selection/parameter selection ==
  data: i input; k output; k_all input; b_all input; l0_all input; b output; l0 output
function [k, b, l0] = parameter_selection(i, k_all, b_all, l0_all)

k=k_all(i);
b=b_all(i);
l0=l0_all(i);

== matlab function tensegrity_Val_like_sim_one_stage_v02/internal cable force_13/cable force/cable force computation ==
  data: k input; Fc output; b input; l0 input; l input; v input
function Fc = cable_force(k, b,l0, l, v)

Fc=k*(l-l0) + b*v;
